simulink model "lab1b"  (R2019b)
settings: Solver=VariableStepAuto  StartTime=0.0  StopTime=10.0  MaxStep=1e-4  RelTol=1e-3
model workspace (MAT data in the model file):
  a = 1
  f = 1
libraries: simulink x1
settings Model: Creator=eisendani  LastModifiedBy=eisendani

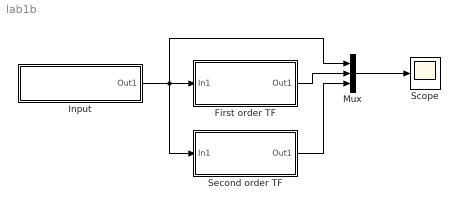
== system lab1b ==
  "First order TF " : Subsystem  mask{a=1}
      mask prompts: a "denominator"
  "Input " : Subsystem  mask{f=3}
      mask prompts: f "function"
  Mux : Mux  Inputs=3
  Scope : Scope
  Second order TF : Subsystem  mask{a=1}
      mask prompts: a "denominator"
  wires:
  "Input "/1(Out1) -> Second order TF/1(In1), Mux/1, "First order TF "/1(In1)
  "First order TF "/1(Out1) -> Mux/2
  Mux/1 -> Scope/1
  Second order TF/1(Out1) -> Mux/3

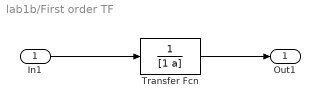
== system lab1b/First order TF  ==
  In1 : Inport
  Transfer Fcn : TransferFcn  Denominator=[1 a]
  Out1 : Outport
  wires:
  In1/1 -> Transfer Fcn/1
  Transfer Fcn/1 -> Out1/1

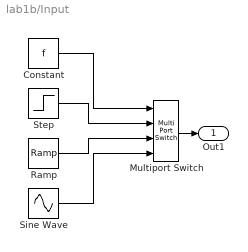
== system lab1b/Input  ==
  Constant : Constant  Value=f
  Multiport Switch : MultiPortSwitch
  Ramp : simulink/Sources/Ramp  slope=1  start=0  InitialOutput=0
  Sine Wave : Sin  Frequency=2*pi  SampleTime=0
  Step : Step  Time=0.5  SampleTime=0
  Out1 : Outport
  wires:
  Sine Wave/1 -> Multiport Switch/4
  Constant/1 -> Multiport Switch/1
  Step/1 -> Multiport Switch/2
  Ramp/1 -> Multiport Switch/3
  Multiport Switch/1 -> Out1/1

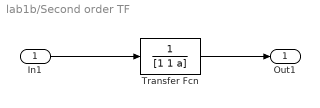
== system lab1b/Second order TF ==
  In1 : Inport
  Transfer Fcn : TransferFcn  Denominator=[1 1 a]
  Out1 : Outport
  wires:
  Transfer Fcn/1 -> Out1/1
  In1/1 -> Transfer Fcn/1
